simulink model "ExamplePedestrian"  (Simulink 9.2)
settings: Solver=FixedStepDiscrete  StartTime=0.0  StopTime=inf  FixedStep=0.001  RelTol=1e-3  EnableMultiTasking=on
libraries: rFproPhysicsLib x9
settings Model: Creator=enewton  LastModifiedBy=SeanKavanagh
settings OptimizationCC: ExpressionDepthLimit=2147483647
settings DebuggingCC: SolverPrmCheckMsg=warning
settings RTWCC: SystemTargetFile=rfpro.tlc  MakeCommand="make_rtw OPTS=\"-DRUN_PHYSICS\""  TemplateMakefile=rfpro.tmf  Description=rFpro Target (Run Physics)  TargetLang=C++
settings STFCustomTargetCC: ModelReferenceCompliant=off  GeneratePreprocessorConditionals=Disable all  CombineOutputUpdateFcns=on  MatFileLogging=on  CPPClassGenCompliant=on  GRTInterface=off  SystemTargetFile=rfpro.tlc
settings GRTTargetCC: ModelReferenceCompliant=off  ParMdlRefBuildCompliant=off  CompOptLevelCompliant=off  ConcurrentExecutionCompliant=off  CombineOutputUpdateFcns=on  GRTInterface=off  UseToolchainInfoCompliant=off

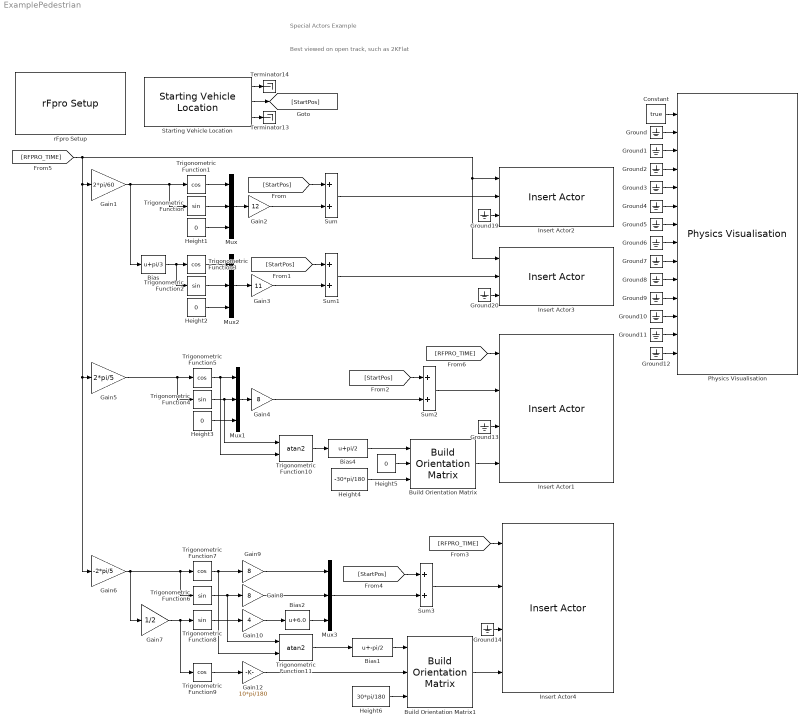
== system ExamplePedestrian ==
  note: Special Actors Example
  note: Best viewed on open track, such as 2KFlat
  Bias : Bias  Bias=pi/3
  Bias1 : Bias  Bias=-pi/2
  Bias2 : Bias  Bias=6.0
  Bias4 : Bias  Bias=pi/2
  Build Orientation Matrix : rFproPhysicsLib/Build Orientation Matrix  ISOAxes=on  YPROrder=on
  Build Orientation Matrix1 : rFproPhysicsLib/Build Orientation Matrix  ISOAxes=on  YPROrder=on
  Constant : Constant  Value=true
  Gain1 : Gain  Gain=2*pi/60
  Gain10 : Gain  Gain=4
  Gain12 : Gain  Gain=10*pi/180
  Gain2 : Gain  Gain=12
  Gain3 : Gain  Gain=11
  Gain4 : Gain  Gain=8
  Gain5 : Gain  Gain=2*pi/5
  Gain6 : Gain  Gain=-2*pi/5
  Gain7 : Gain  Gain=1/2
  Gain8 : Gain  Gain=8
  Gain9 : Gain  Gain=8
  Ground{,1..14,19..20} (17 alike) : Ground
  Height{1..3,5} (4 alike) : Constant  Value=0
  Height4 : Constant  Value=-30*pi/180
  Height6 : Constant  Value=30*pi/180
  Insert Actor1 : rFproPhysicsLib/Insert Actor  actorType='TRF_Moped_Yamaha_Red_01'  instanceName=''  specialType=Motorcycle  doPreLoad=on  headingValid=off  heightValid=off  fixedHeight=0  relHeightFlag=on  orientationValid=on  period=-1  offset=0  useReverseByteOrder=on  rFpro__platform=Remote Model - Default
  Insert Actor2 : rFproPhysicsLib/Insert Actor  actorType='pedestrianJennyB'  instanceName=''  specialType=Pedestrian  doPreLoad=on  headingValid=off  heightValid=off  fixedHeight=0  relHeightFlag=on  orientationValid=off  period=-1  offset=0  useReverseByteOrder=on  rFpro__platform=Remote Model - Default
  Insert Actor3 : rFproPhysicsLib/Insert Actor  actorType='pedestrian01'  instanceName=''  specialType=Pedestrian  doPreLoad=on  headingValid=off  heightValid=off  fixedHeight=0  relHeightFlag=on  orientationValid=off  period=-1  offset=0  useReverseByteOrder=on  rFpro__platform=Remote Model - Default
  Insert Actor4 : rFproPhysicsLib/Insert Actor  actorType='pigeon'  instanceName=''  specialType=Animal  doPreLoad=on  headingValid=off  heightValid=on  fixedHeight=0  relHeightFlag=on  orientationValid=on  period=-1  offset=0  useReverseByteOrder=on  rFpro__platform=Remote Model - Default
  Mux{,1..3} (4 alike) : Mux  Inputs=3
  Physics Visualisation : rFproPhysicsLib/Physics Visualisation  PAR_SKIP_INTERNAL_PHYSICS=off  PAR_ACCEL_VALID=off  PAR_ROT_ACCEL_VALID=off  PAR_GEAR_VALID=off  PAR_RPM_VALID=off  PAR_INPUTS_VALID=on  PAR_STEER_TORQUE_VALID=on  PAR_HEADLIGHTS_ON_VALID=off  PAR_WHEEL_POS_VALID=off  PAR_WHEEL_ORI_VALID=off  PAR_TYRE_PARAMS_VALID=off  PAR_WHEEL_ROTATION_VALID=off  PAR_WHEEL_BRAKE_TEMP_VALID=off  PAR_WHEEL_TREAD_TEMP_VALID=off  PAR_WHEEL_AIR_TEMP_VALID=off  period=-1  offset=0  useReverseByteOrder=on  rFpro__platform=Remote Model - Default
  Starting Vehicle Location : rFproPhysicsLib/Starting Vehicle Location  cg_offset=[0, 0, 0]  numPackets=1  rFpro__platform=Remote Model - Default
  Sum{,1..3} (4 alike) : Sum
  Terminator13 : Terminator
  Terminator14 : Terminator
  Trigonometric Function{,2,4,6,8} (5 alike) : Trigonometry
  Trigonometric Function{1,3,5,7,9} (5 alike) : Trigonometry  Operator=cos
  Trigonometric Function10 : Trigonometry  Operator=atan2
  Trigonometric Function11 : Trigonometry  Operator=atan2
  rFpro Setup : rFproPhysicsLib/rFpro Setup  platform=Remote Model - Default  stopOnSessionEnd=on  usePseudoRealtime=on  syncToRF=on  useReverseByteOrder=off  useRfTime=on  minIterations=4  maxIterations=1000  ipReceiveAddress='127.0.0.1'  ipReceivePort=11054  receiveSampleTime=-1  ipTransmitAddress='127.0.0.1'  ipTransmitPort=11052  transmitSampleTime=-1  pluginType=RUN_PHYSICS  sysTarget=xpctarget.tlc  templateMakeFile=xpc_default_tmf  makeCommand=make_rtw  buildDesc=xPC target
  wires:
  Constant/1 -> Physics Visualisation/1
  Ground/1 -> Physics Visualisation/2
  Ground1/1 -> Physics Visualisation/3
  Ground2/1 -> Physics Visualisation/4
  Ground3/1 -> Physics Visualisation/5
  Ground4/1 -> Physics Visualisation/6
  Ground5/1 -> Physics Visualisation/7
  Ground6/1 -> Physics Visualisation/8
  Ground7/1 -> Physics Visualisation/9
  Ground8/1 -> Physics Visualisation/10
  Ground9/1 -> Physics Visualisation/11
  Ground10/1 -> Physics Visualisation/12
  Ground11/1 -> Physics Visualisation/13
  Ground12/1 -> Physics Visualisation/14
  Starting Vehicle Location/3 -> Terminator13/1
  Starting Vehicle Location/1 -> Terminator14/1
  [RFPRO_TIME] -> Insert Actor3/1, Insert Actor2/1, Gain6/1, Gain5/1, Gain1/1
  Gain1/1 -> Bias/1, Trigonometric Function/1, Trigonometric Function1/1
  Bias/1 -> Trigonometric Function2/1, Trigonometric Function3/1
  Trigonometric Function/1 -> Mux/2
  Height1/1 -> Mux/3
  Trigonometric Function1/1 -> Mux/1
  Height2/1 -> Mux2/3
  Trigonometric Function2/1 -> Mux2/2
  Trigonometric Function3/1 -> Mux2/1
  Ground19/1 -> Insert Actor2/3
  Ground20/1 -> Insert Actor3/3
  Sum/1 -> Insert Actor2/2
  Sum1/1 -> Insert Actor3/2
  Mux/1 -> Gain2/1
  Mux2/1 -> Gain3/1
  Gain2/1 -> Sum/2
  Gain3/1 -> Sum1/2
  Height3/1 -> Mux1/3
  Trigonometric Function4/1 -> Trigonometric Function10/1, Mux1/2
  Trigonometric Function5/1 -> Trigonometric Function10/2, Mux1/1
  Sum2/1 -> Insert Actor1/2
  Mux1/1 -> Gain4/1
  Gain4/1 -> Sum2/2
  Gain5/1 -> Trigonometric Function4/1, Trigonometric Function5/1
  Height5/1 -> Build Orientation Matrix/2
  Height4/1 -> Build Orientation Matrix/3
  Starting Vehicle Location/2 -> [StartPos]
  [StartPos] -> Sum/1
  [StartPos] -> Sum1/1
  [StartPos] -> Sum2/1
  Gain6/1 -> Gain7/1, Trigonometric Function6/1, Trigonometric Function7/1
  Gain7/1 -> Trigonometric Function9/1, Trigonometric Function8/1
  Trigonometric Function9/1 -> Gain12/1
  Trigonometric Function7/1 -> Trigonometric Function11/2, Gain9/1
  Trigonometric Function6/1 -> Trigonometric Function11/1, Gain8/1
  Gain10/1 -> Bias2/1
  Gain8/1 -> Mux3/2
  Bias2/1 -> Mux3/3
  Mux3/1 -> Sum3/2
  [RFPRO_TIME] -> Insert Actor4/1
  Ground14/1 -> Insert Actor4/3
  Height6/1 -> Build Orientation Matrix1/3
  Gain12/1 -> Build Orientation Matrix1/2
  [StartPos] -> Sum3/1
  Sum3/1 -> Insert Actor4/2
  Gain9/1 -> Mux3/1
  Trigonometric Function10/1 -> Bias4/1
  Build Orientation Matrix/1 -> Insert Actor1/4
  Bias4/1 -> Build Orientation Matrix/1
  Trigonometric Function8/1 -> Gain10/1
  Trigonometric Function11/1 -> Bias1/1
  Bias1/1 -> Build Orientation Matrix1/1
  Build Orientation Matrix1/1 -> Insert Actor4/4
  Ground13/1 -> Insert Actor1/3
  [RFPRO_TIME] -> Insert Actor1/1
